simulink model "M1"  (R2015b)
settings: Solver=VariableStepAuto  StartTime=-10  StopTime=10.0  RelTol=1e-3
libraries: simulink x1
settings Model: Creator=Pouya  LastModifiedBy=Pouya

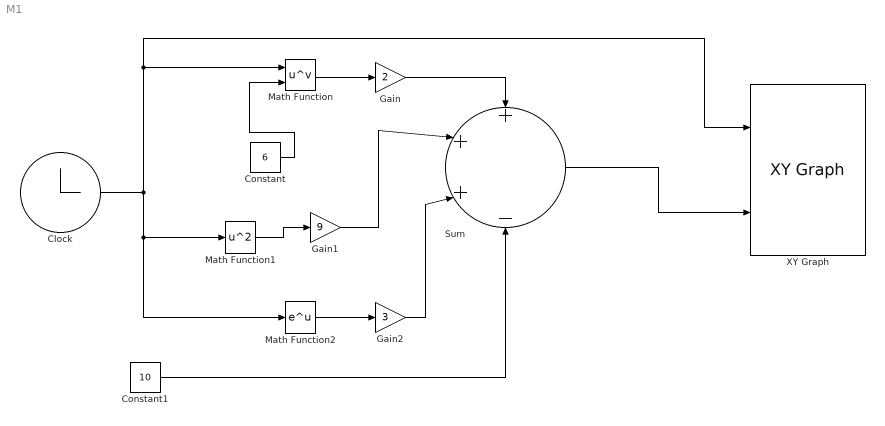
== system M1 ==
  Clock : Clock
  Constant : Constant  Value=6
  Constant1 : Constant  Value=10
  Gain : Gain  Gain=2
  Gain1 : Gain  Gain=9
  Gain2 : Gain  Gain=3
  Math Function : Math  Operator=pow  SaturateOnIntegerOverflow=on
  Math Function1 : Math  Operator=square  SaturateOnIntegerOverflow=on
  Math Function2 : Math  SaturateOnIntegerOverflow=on
  Sum : Sum  Inputs=+++-
  XY Graph : simulink/Sinks/XY Graph  xmin=-10  xmax=10  ymin=-100  ymax=100  st=-1
  wires:
  Constant/1 -> Math Function/2
  Clock/1 -> Math Function/1, XY Graph/1, Math Function2/1, Math Function1/1
  Constant1/1 -> Sum/4
  Sum/1 -> XY Graph/2
  Math Function/1 -> Gain/1
  Gain/1 -> Sum/1
  Math Function1/1 -> Gain1/1
  Gain1/1 -> Sum/2
  Math Function2/1 -> Gain2/1
  Gain2/1 -> Sum/3
